simulink model "Series_Balancing"  (R2024b)
settings: Solver=FixedStepAuto  StartTime=0.0  StopTime=30  FixedStep=0.0001  RelTol=1e-3
model workspace (MAT data in the model file):
  Deg2Rad = 0.0174533
  Rad2Deg = 57.2957795
values from neighbouring files (symbols this model uses):
  D = zeros(6,2)    [old_Lqr_matrix.m]
  K = lqr(sys, Q, R)    [old_Lqr_matrix.m]
  X = [theta(t); theta_dot; x(t); x_dot; phi(t); phi_dot]    [old_Lqr_matrix.m]
undefined symbols (not defined in the file or in its folder): L0, Y, Z
libraries: sm_lib x47, nesl_utility x22, slpidlib x4
(part 1 of 3)
settings Model: Creator=Brownlm1  LastModifiedBy=Chen

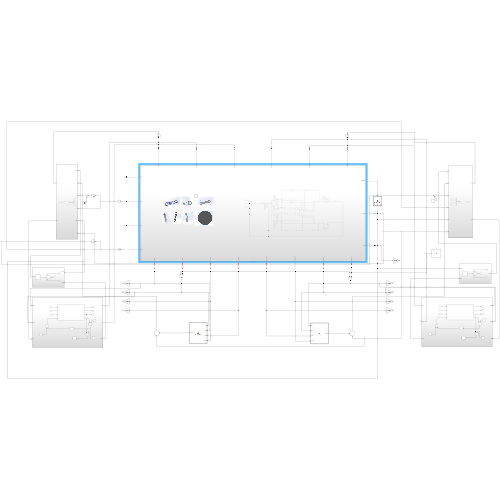
[thumbnail: Simulink's stored preview of the top-level diagram]
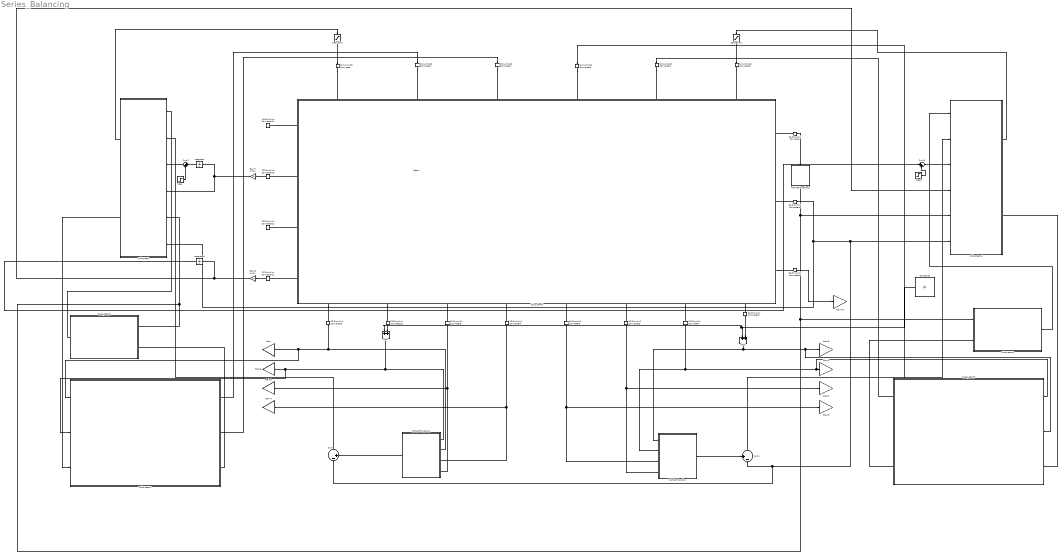
== system Series_Balancing ==
  Add1 : Sum  Inputs=+|+
  Add2 : Sum  Inputs=+|+
  Constant2 : Constant  Value=pi
  Gain{,1..6,8,16} (9 alike) : Gain  Gain=Rad2Deg
  Gain7 : Gain  Gain=0.064
  Gain9 : Gain  Gain=0.064
  Integrator : Integrator
  Integrator1 : Integrator
  MATLAB Function : MATLAB Function  TreatAsAtomicUnit=on
  MATLAB Function1 : MATLAB Function  TreatAsAtomicUnit=on
  MATLAB Function2 : MATLAB Function  TreatAsAtomicUnit=on
  PS-Simulink Converter{,1..14} (15 alike) : nesl_utility/PS-Simulink Converter  PhysicalDomain=network_engine_domain  SubClassName=ps_output  LeftPortType=input  RightPortType=output  PseudoPeriodic=off  Frequencies=[]  VectorFormat=inherit  Unit=inherit  AffineConversion=off
  Saturation : Saturate  UpperLimit=2  LowerLimit=-2
  Saturation1 : Saturate  UpperLimit=2  LowerLimit=-2
  Simulink-PS Converter{,1..5} (6 alike) : nesl_utility/Simulink-PS Converter  PhysicalDomain=network_engine_domain  SubClassName=ps_input  LeftPortType=input  RightPortType=output  PseudoPeriodic=off  Frequencies=[]  NoiseDistribution=none  NoiseParameters=[]  Unit=1  AffineConversion=off  FilteringAndDerivatives=provide  SimscapeFilterOrder=1  InputFilterTimeConstant=0.001  UdotUserProvided=0
  Step : Step  Time=3  After=-1  SampleTime=0
  Step1 : Step  Time=3  After=-1  SampleTime=0
  Step2 : Step  Time=3  After=-1  SampleTime=0
  Subsystem : Subsystem
  Subsystem1 : Subsystem
  Subsystem2 : Subsystem
      settings: PortSchema="{\"entries\":[{\"content\":{\"sides\":[{\"content\":{\"connectorIds\":[\"LConn1\",\"LConn2\",\"LConn3\",\"LConn4\"]},\"type\":\"ConnectorPlacement.EquallySpacedRectSide\",\"uuid\":\"241f321a-7666-4cba-8665-095b31e601a6\"},{\"content\":{\"connectorIds\":[\"RConn1\",\"RConn2\",\"RConn3\"],\"side\":\"RIGHT\"},\"type\":\"ConnectorPlacement.EquallySpacedRectSide\",\"uuid\":\"d9e9ebe8-43ef-42e8-942a-696afc462c17\"},{\"content\":{\"connectorIds\":[\"LConn5\",\"LConn6\",\"LConn7\",\"LConn8\",\"LConn9\",\"LConn10\"],\"side\":\"TOP\"},\"type\":\"ConnectorPlacement.EquallySpacedRectSide\",\"uuid\":\"aa23ff5a-3d8e-4891-9c0d-f07b06494546\"},{\"content\":{\"connectorIds\":[\"RConn4\",\"RConn5\",\"RConn6\",\"RConn7\",\"RConn8\",\"RConn9\",\"RConn10\",\"RConn11\"],\"side\":\"BOTTOM\"},\"type\":\"ConnectorPlacement.EquallySpacedRectSide\",\"uuid\":\"21f405dc-d0f9-4592-af84-06e12d3506cf\"}]},\"type\":\"ConnectorPlacement.EquallySpacedConnector\",\"uuid\":\"3f989f65-e7d0-461e-bbf8-8f2cad2f1b46\"}],\"packageUris\":[\"http://schema.mathworks.com/mf0/Connector/R2020b\"],\"version\":\"1.0\"}"
  Subsystem3 : Subsystem
  Subsystem4 : Subsystem
  Subsystem5 : Subsystem
  Subsystem6 : Subsystem
  Sum : Sum  Inputs=|-+
  Sum1 : Sum  Inputs=+-|
  Sum2 : Sum  Inputs=|++
  Sum3 : Sum  Inputs=|++
  wires:
  PS-Simulink Converter10/1 -> Add1/2
  PS-Simulink Converter3/1 -> MATLAB Function1/4(d_phi4), Gain5/1
  PS-Simulink Converter4/1 -> MATLAB Function1/3(d_phi1), Gain4/1
  PS-Simulink Converter6/1 -> MATLAB Function/4(d_phi4), Gain2/1
  PS-Simulink Converter8/1 -> Add2/2
  Add1/1 -> Gain6/1, Subsystem4/2(phi1), MATLAB Function1/1(phi1)
  Constant2/1 -> Add2/1, Add1/1
  PS-Simulink Converter9/1 -> Subsystem4/1(phi4), Gain/1, MATLAB Function1/2(phi4)
  Add2/1 -> Subsystem5/2(phi1), Gain8/1, MATLAB Function/1(phi1)
  Subsystem4/1(T2) -> Simulink-PS Converter4/1
  Subsystem4/2(T1) -> Simulink-PS Converter1/1
  PS-Simulink Converter7/1 -> Subsystem5/1(phi4), Gain1/1, MATLAB Function/2(phi4)
  Subsystem5/1(T2) -> Simulink-PS Converter2/1
  PS-Simulink Converter11/1 -> Gain9/1
  PS-Simulink Converter2/1 -> Gain16/1
  PS-Simulink Converter/1 -> MATLAB Function2/1(q)
  MATLAB Function2/2(pitch) -> Subsystem6/1(pitch), Subsystem/5(pitch), Subsystem3/1(pitch), Subsystem1/5(In5)
  Subsystem4/3(phi0) -> Subsystem3/2(phi0)
  Subsystem5/3(phi0) -> Subsystem6/2(phi0)
  Subsystem3/1(theta) -> Subsystem/1(theta)
  Subsystem6/1(theta) -> Subsystem1/1(In1)
  PS-Simulink Converter5/1 -> MATLAB Function/3(d_phi1), Gain3/1
  MATLAB Function1/1(d_phi0) -> Sum/2
  MATLAB Function/1(d_phi0) -> Sum1/1
  PS-Simulink Converter1/1 -> Sum/1, Sum1/2, Subsystem1/6(In6), Subsystem/6(In6)
  Sum/1 -> Subsystem/2(In2)
  Sum1/1 -> Subsystem1/2(In2)
  Subsystem5/2(T1) -> Simulink-PS Converter3/1
  Subsystem/1(T) -> Saturation/1
  Subsystem1/1(T) -> Saturation1/1
  Saturation/1 -> Simulink-PS Converter/1
  Saturation1/1 -> Simulink-PS Converter5/1
  Subsystem1/2(Tp) -> Subsystem5/3(Tp)
  Subsystem/2(Tp) -> Subsystem4/3(Tp)
  PS-Simulink Converter13/1 -> Gain7/1
  Gain7/1 -> Integrator/1, Subsystem/4(In4)
  Gain9/1 -> Integrator1/1, Subsystem1/4(In4)
  Integrator1/1 -> Sum3/1
  Integrator/1 -> Sum2/1
  Sum2/1 -> Subsystem/3(In3)
  Step/1 -> Sum2/2
  Sum3/1 -> Subsystem1/3(In3)
  Step2/1 -> Sum3/2
  connections:
  PS-Simulink Converter/LConn1 -- Subsystem2/RConn1
  PS-Simulink Converter1/LConn1 -- Subsystem2/RConn2
  Subsystem2/RConn3 -- PS-Simulink Converter2/LConn1
  PS-Simulink Converter3/LConn1 -- Subsystem2/RConn6
  PS-Simulink Converter4/LConn1 -- Subsystem2/RConn7
  PS-Simulink Converter5/LConn1 -- Subsystem2/RConn8
  PS-Simulink Converter6/LConn1 -- Subsystem2/RConn9
  Subsystem2/RConn10 -- PS-Simulink Converter7/LConn1
  Subsystem2/RConn11 -- PS-Simulink Converter8/LConn1
  Subsystem2/RConn5 -- PS-Simulink Converter10/LConn1
  Subsystem2/RConn4 -- PS-Simulink Converter9/LConn1
  Simulink-PS Converter/RConn1 -- Subsystem2/LConn5
  Simulink-PS Converter4/RConn1 -- Subsystem2/LConn6
  Simulink-PS Converter1/RConn1 -- Subsystem2/LConn7
  Simulink-PS Converter3/RConn1 -- Subsystem2/LConn8
  Simulink-PS Converter2/RConn1 -- Subsystem2/LConn9
  Simulink-PS Converter5/RConn1 -- Subsystem2/LConn10
  Subsystem2/LConn1 -- PS-Simulink Converter14/LConn1
  Subsystem2/LConn2 -- PS-Simulink Converter13/LConn1
  Subsystem2/LConn3 -- PS-Simulink Converter12/LConn1
  Subsystem2/LConn4 -- PS-Simulink Converter11/LConn1

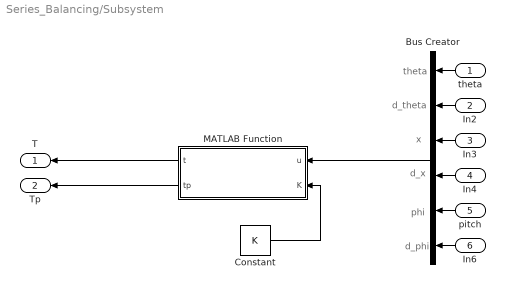
== system Series_Balancing/Subsystem ==
  note: theta
  note: d_theta
  note: x
  note: d_x
  note: phi
  note: d_phi
  theta : Inport
  In2 : Inport  Port=2
  In3 : Inport  Port=3
  In4 : Inport  Port=4
  pitch : Inport  Port=5
  In6 : Inport  Port=6
  Bus Creator : BusCreator  Inputs=6
  Constant : Constant  Value=K
  MATLAB Function : MATLAB Function  TreatAsAtomicUnit=on
  T : Outport
  Tp : Outport  Port=2
  wires:
  In6/1 -> Bus Creator/6
  In2/1 -> Bus Creator/2
  In4/1 -> Bus Creator/4
  In3/1 -> Bus Creator/3
  theta/1 -> Bus Creator/1
  pitch/1 -> Bus Creator/5
  Bus Creator/1 -> MATLAB Function/1(u)
  MATLAB Function/1(t) -> T/1
  MATLAB Function/2(tp) -> Tp/1
  Constant/1 -> MATLAB Function/2(K)

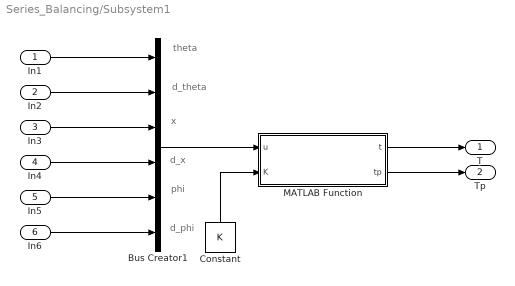
== system Series_Balancing/Subsystem1 ==
  note: d_phi
  note: phi
  note: d_x
  note: d_theta
  note: x
  note: theta
  In1 : Inport
  In2 : Inport  Port=2
  In3 : Inport  Port=3
  In4 : Inport  Port=4
  In5 : Inport  Port=5
  In6 : Inport  Port=6
  Bus Creator1 : BusCreator  Inputs=6
  Constant : Constant  Value=K
  MATLAB Function : MATLAB Function  TreatAsAtomicUnit=on
  T : Outport
  Tp : Outport  Port=2
  wires:
  In1/1 -> Bus Creator1/1
  In5/1 -> Bus Creator1/5
  In6/1 -> Bus Creator1/6
  In2/1 -> Bus Creator1/2
  Bus Creator1/1 -> MATLAB Function/1(u)
  MATLAB Function/1(t) -> T/1
  MATLAB Function/2(tp) -> Tp/1
  Constant/1 -> MATLAB Function/2(K)
  In3/1 -> Bus Creator1/3
  In4/1 -> Bus Creator1/4
